simulink model "fim_tg"  (R2018a)
settings: Solver=VariableStepAuto  StartTime=0.0  StopTime=1000  RelTol=1e-3
values from neighbouring files (symbols this model uses):
  A = zeros(nz*nr + 1)    [teste1_7_aberto_2.m]
  B = zeros(nr*nz + 1, 1)    [teste1_7_aberto_2.m]
  C = repelem(0,1, nz*nr + 1)    [teste1_7_aberto_2.m]
settings Model: Creator=jp021996  LastModifiedBy=cgaa1

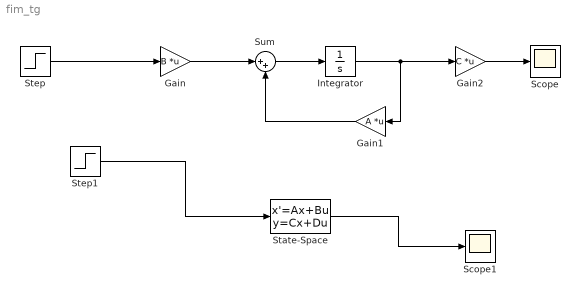
== system fim_tg ==
  Gain : Gain  Gain=B  Multiplication=Matrix(K*u)
  Gain1 : Gain  Gain=A  Multiplication=Matrix(K*u) (u vector)
  Gain2 : Gain  Gain=C  Multiplication=Matrix(K*u) (u vector)
  Integrator : Integrator  InitialCondition=0.4
  Scope : Scope
  Scope1 : Scope
  State-Space : StateSpace  A=A  B=B  C=C  D=0  InitialCondition=0.4
  Step : Step  Time=0  SampleTime=0
  Step1 : Step  Time=0  SampleTime=0
  Sum : Sum  Inputs=|++
  wires:
  Step/1 -> Gain/1
  Gain/1 -> Sum/1
  Gain2/1 -> Scope/1
  Sum/1 -> Integrator/1
  Step1/1 -> State-Space/1
  State-Space/1 -> Scope1/1
  Integrator/1 -> Gain1/1, Gain2/1
  Gain1/1 -> Sum/2
